simulink model "NEW_SINGLE_DANBAI"  (Simulink 7.4)
settings: Solver=ode45  StartTime=0.0  StopTime=10.0  RelTol=1e-3
undefined symbols (not defined in the file): RootGround, RootPart
libraries: mblibv1 x8
settings Model: Creator=zmtaishiji
settings SimMechanicsCC: VisOnUpdateDiagram=on  VisDuringSimulation=on

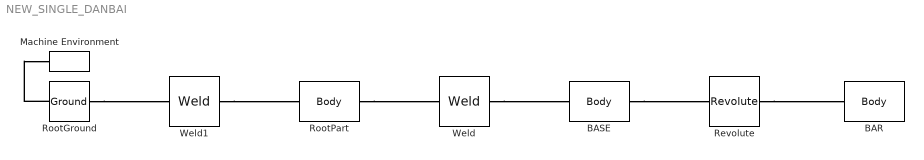
== system NEW_SINGLE_DANBAI ==
  BAR : mblibv1/Bodies/Body  DialogController=MECH.DynMechDlgSource  PhysicalDomain=mechanical  SubClassName=Unknown  LeftPortType=workingframe  RightPortType=workingframe  LConnTagsString=CS2  PMImportedID=40  UpdateFromCAD=on  DialogClass=MechanicalBodyBlock  Mass=6.65597e+008  MassUnits=kg  InertiaUnits=kg*m^2  Inertia=[7.43264e+006,0,0;0,7.41741e+006,0;0,0,202136]  Shape=Cylinder  ShapeDims=[1 1]  ShapeUnits=m  ShapeUse=false  Density=1  DensityUnits=kg/m^3  DensityUse=false  GraphicsMode=GFXFILE  GraphicsFileName=BAR_prt.stl  BodyColorSelMode=COLORPALETTE  BodyColor=[0;1;0]  AttachedToCS=CS1  CG=Right$CG$[135.181 57.5 -215.507]$WORLD$WORLD$mm$[0 -0.79224 -0.610209;1 0 0;0 -0.610209 0.79224]$3x3 Transform$rad$WORLD$false$40::CG(AUTOGEN)  WorkingFrames=Right$CS1$[149.501 57.5 -234.099]$WORLD$WORLD$mm$[0 -0.79224 -0.610209;1 0 0;0 -0.610209 0.79224]$3x3 Transform$rad$WORLD$false$40::CS1(AUTOGEN)#Left$CS2$[0 50 -40]$WORLD$WORLD$mm$[1 0 0;0 1 0;0 0 1]$3x3 Transform$rad$WORLD$true$39:-:40::40(AUTOGEN)  CGPos=[135.181 57.5 -215.507]  CGRot=[0 -0.79224 -0.610209;1 0 0;0 -0.610209 0.79224]  CS0Pos=[]  CS0Rot=[]  CS1Pos=[149.501 57.5 -234.099]  CS1Rot=[0 -0.79224 -0.610209;1 0 0;0 -0.610209 0.79224]  CS2Pos=[0 50 -40]  CS2Rot=[1 0 0;0 1 0;0 0 1]  CS3Pos=[]  CS3Rot=[]  CS4Pos=[]  CS4Rot=[]  CS5Pos=[]  CS5Rot=[]  CS6Pos=[]  CS6Rot=[]  CS7Pos=[]  CS7Rot=[]  CS8Pos=[]  CS8Rot=[]  CS9Pos=[]  CS9Rot=[]  CS10Pos=[]  CS10Rot=[]  CS11Pos=[]  CS11Rot=[]  CS12Pos=[]  CS12Rot=[]  CS13Pos=[]  CS13Rot=[]  CS14Pos=[]  CS14Rot=[]  CS15Pos=[]  CS15Rot=[]  CS16Pos=[]  CS16Rot=[]  CS17Pos=[]  CS17Rot=[]  CS18Pos=[]  CS18Rot=[]  CS19Pos=[]  CS19Rot=[]  CS20Pos=[]  CS20Rot=[]
  BASE : mblibv1/Bodies/Body  DialogController=MECH.DynMechDlgSource  PhysicalDomain=mechanical  SubClassName=Unknown  LeftPortType=workingframe  RightPortType=workingframe  LConnTagsString=CS3  RConnTagsString=CS2  PMImportedID=39  UpdateFromCAD=on  DialogClass=MechanicalBodyBlock  Mass=2.76822e+008  MassUnits=kg  InertiaUnits=kg*m^2  Inertia=[384703,0,0;0,352039,92335.7;0,92335.7,504054]  Shape=Cylinder  ShapeDims=[1 1]  ShapeUnits=m  ShapeUse=false  Density=1  DensityUnits=kg/m^3  DensityUse=false  GraphicsMode=GFXFILE  GraphicsFileName=BASE_prt.stl  BodyColorSelMode=COLORPALETTE  BodyColor=[0.11;0.11;0.11]  AttachedToCS=CS1  CG=Right$CG$[0 11.7943 -10.863]$WORLD$WORLD$mm$[1 0 0;0 1 0;0 0 1]$3x3 Transform$rad$WORLD$false$39::CG(AUTOGEN)  WorkingFrames=Right$CS1$[0 0 0]$WORLD$WORLD$mm$[1 0 0;0 1 0;0 0 1]$3x3 Transform$rad$WORLD$false$39::CS1(AUTOGEN)#Right$CS2$[0 50 -40]$WORLD$WORLD$mm$[1 0 0;0 1 0;0 0 1]$3x3 Transform$rad$WORLD$true$39:-:40::39(AUTOGEN)#Left$CS3$[95.4735 44.0746 -155.396]$WORLD$WORLD$mm$[1 0 0;0 1 0;0 0 1]$3x3 Transform$rad$WORLD$true$:-:39::39(AUTOGEN)  CGPos=[0 11.7943 -10.863]  CGRot=[1 0 0;0 1 0;0 0 1]  CS0Pos=[]  CS0Rot=[]  CS1Pos=[0 0 0]  CS1Rot=[1 0 0;0 1 0;0 0 1]  CS2Pos=[0 50 -40]  CS2Rot=[1 0 0;0 1 0;0 0 1]  CS3Pos=[95.4735 44.0746 -155.396]  CS3Rot=[1 0 0;0 1 0;0 0 1]  CS4Pos=[]  CS4Rot=[]  CS5Pos=[]  CS5Rot=[]  CS6Pos=[]  CS6Rot=[]  CS7Pos=[]  CS7Rot=[]  CS8Pos=[]  CS8Rot=[]  CS9Pos=[]  CS9Rot=[]  CS10Pos=[]  CS10Rot=[]  CS11Pos=[]  CS11Rot=[]  CS12Pos=[]  CS12Rot=[]  CS13Pos=[]  CS13Rot=[]  CS14Pos=[]  CS14Rot=[]  CS15Pos=[]  CS15Rot=[]  CS16Pos=[]  CS16Rot=[]  CS17Pos=[]  CS17Rot=[]  CS18Pos=[]  CS18Rot=[]  CS19Pos=[]  CS19Rot=[]  CS20Pos=[]  CS20Rot=[]
  Machine Environment : mblibv1/Bodies/Machine Environment  DialogController=MECH.DialogSource  SystemSampleTime=-1  PortType=env  PhysicalDomain=Mechanical  DialogTemplateClass=MECH.MachineEnvironment  SyncWhenCopied=off  Gravity=[0 -9.81 0]  GravityUnits=m/s^2  GravityAsSignal=off  Dimensionality=Auto-detect  AnalysisType=Forward dynamics  LinearAssemblyTolerance=1e-3  LinearAssemblyToleranceUnits=m  AngularAssemblyTolerance=1e-3  AngularAssemblyToleranceUnits=rad  ConstraintSolverType=Stabilizing  ConstraintRelTolerance=1e-4  ConstraintAbsTolerance=1e-4  UseRobustSingularityHandling=off  RedundancyAnalysisToleranceType=Automatically select tolerance  RedundancyAnalysisTolerance=1e-14  StatePerturbationType=Fixed  PerturbationSize=1e-5  VisualizeMachine=on  BodyVisualizationType=Use model default body geometries  BodyColorSelMode=Use model default  DefaultBodyColor=[1 0 0]
  Revolute : mblibv1/Joints/Revolute  DialogController=MECH.DynMechDlgSource  PhysicalDomain=mechanical  SubClassName=Unknown  LeftPortType=blob  RightPortType=blob  LConnTagsString=__newl0  RConnTagsString=__newr0  PMImportedID=39:-:40  UpdateFromCAD=on  NumSAPorts=0  CutJoint=off  MarkAsCut=off  Primitives=prismatic  PrimitiveProps=R1$WORLD$[0,-1,0]$revolute  DialogClass=JointBlock  R1Axis=[0,-1,0]
  RootGround : mblibv1/Bodies/Ground  DialogController=MECH.DynMechDlgSource  SystemSampleTime=-1  PMImportedID=RootGround  UpdateFromCAD=on  LeftPortType=env  RightPortType=workingframe  PhysicalDomain=Mechanical  DialogClass=GroundBlock  CoordPosition=[95.4735,44.0746,-155.396]  CoordPositionUnits=mm  StateVectorMgrId=-1  MachineId=[0 0]  ShowEnvPort=on
  RootPart : mblibv1/Bodies/Body  DialogController=MECH.DynMechDlgSource  PhysicalDomain=mechanical  SubClassName=Unknown  LeftPortType=workingframe  RightPortType=workingframe  LConnTagsString=CS3  RConnTagsString=CS2  PMImportedID=RootPart  UpdateFromCAD=on  DialogClass=MechanicalBodyBlock  Mass=0  MassUnits=kg  InertiaUnits=kg*m^2  Inertia=[0,0,0;0,0,0;0,0,0]  Shape=Cylinder  ShapeDims=[1 1]  ShapeUnits=m  ShapeUse=false  Density=1  DensityUnits=kg/m^3  DensityUse=false  GraphicsMode=MACHINE_DEFAULT  BodyColorSelMode=MACHINE_DEFAULT  BodyColor=[1 0 0]  AttachedToCS=CS1  CG=Right$CG$[95.4735 44.0746 -155.396]$WORLD$WORLD$mm$[1 0 0;0 1 0;0 0 1]$3x3 Transform$rad$WORLD$false$RootPart::CG(AUTOGEN)  WorkingFrames=Right$CS1$[0 0 0]$WORLD$WORLD$mm$[1 0 0;0 1 0;0 0 1]$3x3 Transform$rad$WORLD$false$RootPart::CS1(AUTOGEN)#Right$CS2$[95.4735 44.0746 -155.396]$WORLD$WORLD$mm$[1 0 0;0 1 0;0 0 1]$3x3 Transform$rad$WORLD$true$:-:39::RootPart(AUTOGEN)#Left$CS3$[95.4735 44.0746 -155.396]$WORLD$WORLD$mm$[1 0 0;0 1 0;0 0 1]$3x3 Transform$rad$WORLD$true$RootGround:-:RootPart::RootPart(AUTOGEN)  CGPos=[95.4735 44.0746 -155.396]  CGRot=[1 0 0;0 1 0;0 0 1]  CS0Pos=[]  CS0Rot=[]  CS1Pos=[0 0 0]  CS1Rot=[1 0 0;0 1 0;0 0 1]  CS2Pos=[95.4735 44.0746 -155.396]  CS2Rot=[1 0 0;0 1 0;0 0 1]  CS3Pos=[95.4735 44.0746 -155.396]  CS3Rot=[1 0 0;0 1 0;0 0 1]  CS4Pos=[]  CS4Rot=[]  CS5Pos=[]  CS5Rot=[]  CS6Pos=[]  CS6Rot=[]  CS7Pos=[]  CS7Rot=[]  CS8Pos=[]  CS8Rot=[]  CS9Pos=[]  CS9Rot=[]  CS10Pos=[]  CS10Rot=[]  CS11Pos=[]  CS11Rot=[]  CS12Pos=[]  CS12Rot=[]  CS13Pos=[]  CS13Rot=[]  CS14Pos=[]  CS14Rot=[]  CS15Pos=[]  CS15Rot=[]  CS16Pos=[]  CS16Rot=[]  CS17Pos=[]  CS17Rot=[]  CS18Pos=[]  CS18Rot=[]  CS19Pos=[]  CS19Rot=[]  CS20Pos=[]  CS20Rot=[]
  Weld : mblibv1/Joints/Weld  DialogController=MECH.DynMechDlgSource  PhysicalDomain=mechanical  SubClassName=Unknown  LeftPortType=blob  RightPortType=blob  LConnTagsString=__newl0  RConnTagsString=__newr0  PMImportedID=:-:39  UpdateFromCAD=on  NumSAPorts=0  CutJoint=off  MarkAsCut=off  Primitives=weld  PrimitiveProps=W$WORLD$[0.57735,0.57735,0.57735]$weld  DialogClass=JointBlock  WAxis=[0.57735,0.57735,0.57735]
  Weld1 : mblibv1/Joints/Weld  DialogController=MECH.DynMechDlgSource  PhysicalDomain=mechanical  SubClassName=Unknown  LeftPortType=blob  RightPortType=blob  LConnTagsString=__newl0  RConnTagsString=__newr0  PMImportedID=RootGround:-:RootPart  UpdateFromCAD=on  NumSAPorts=0  CutJoint=off  MarkAsCut=off  Primitives=weld  PrimitiveProps=W$WORLD$[0.57735,0.57735,0.57735]$weld  DialogClass=JointBlock  WAxis=[0.57735,0.57735,0.57735]
  connections:
  BASE/RConn1 -- Revolute/LConn1
  Revolute/RConn1 -- BAR/LConn1
  RootPart/RConn1 -- Weld/LConn1
  Weld/RConn1 -- BASE/LConn1
  RootGround/RConn1 -- Weld1/LConn1
  Weld1/RConn1 -- RootPart/LConn1
  RootGround/LConn1 -- Machine Environment/RConn1
